simulink model "DigitalControl"  (R2026b)
settings: Solver=VariableStepAuto  MaxStep=0.1  EnableMultiTasking=on
undefined symbols (not defined in the file): deltat, deltat1, DiscIntNeverNeededParam, fden, fnum, Ka, Kf, Ki, Kq, Tal, Ts, W1, W2
libraries: simulink x1
settings Model: DataDictionary=controller.sldd  FPTRunName=Active  ModifiedByFormat=The MathWorks Inc.  Creator=The MathWorks, Inc.  LastModifiedBy=The MathWorks Inc.
settings DataIOCC: LimitDataPoints=on  ReturnWorkspaceOutputs=off  SaveFormat=Array  SaveOutput=off  SaveTime=off  SignalLogging=off  SignalLoggingName=DigitalControl
settings OptimizationCC: LifeSpan=inf  MemsetInitFltsAndDblsToZero=off
settings DebuggingCC: AllowSymbolicDim=off  ArithmeticOperatorsInVariantConditions=warning  FcnCallInpInsideContextMsg=warning  MergeDetectMultiDrivingBlocksExec=none  MultiTaskCondExecSysMsg=none  MultiTaskDSMMsg=warning  SFExecutionAtInitializationDiag=none  SFNoUnconditionalDefaultTransitionDiag=warning  SFUnexpectedBacktrackingDiag=warning  SaveWithParameterizedLinksMsg=none  SignalResolutionControl=TryResolveAllWithWarning  SolverPrmCheckMsg=warning  StateNameClashWarn=warning  UnderspecifiedInitializationDetection=Classic
settings HardwareCC: ProdEndianess=Unspecified  ProdHWDeviceType=32-bit Generic  ProdIntDivRoundTo=Undefined  ProdLargestAtomicFloat=None
settings ModelReferenceCC: ModelReferenceMinAlgLoopOccurrences=on  PropagateSignalLabelsOutOfModel=off
settings SFSimCC: CustomCodeUndefinedFunction=UseInterfaceOnly  SimUseLocalCustomCode=off
settings RTWCC: RTWUseLocalCustomCode=off
settings CodeAppCC: StateflowObjectComments=on
settings GRTTargetCC: CombineOutputUpdateFcns=off  GRTInterface=on  TargetFcnLib=ansi_tfl_tmw.mat  TargetLangStandard=C89/C90 (ANSI)
settings ConfigComp: CovExternalEMLEnable=off  CovSFcnEnable=off  CovSaveCumulativeToWorkspaceVar=on  CovSaveSingleToWorkspaceVar=on

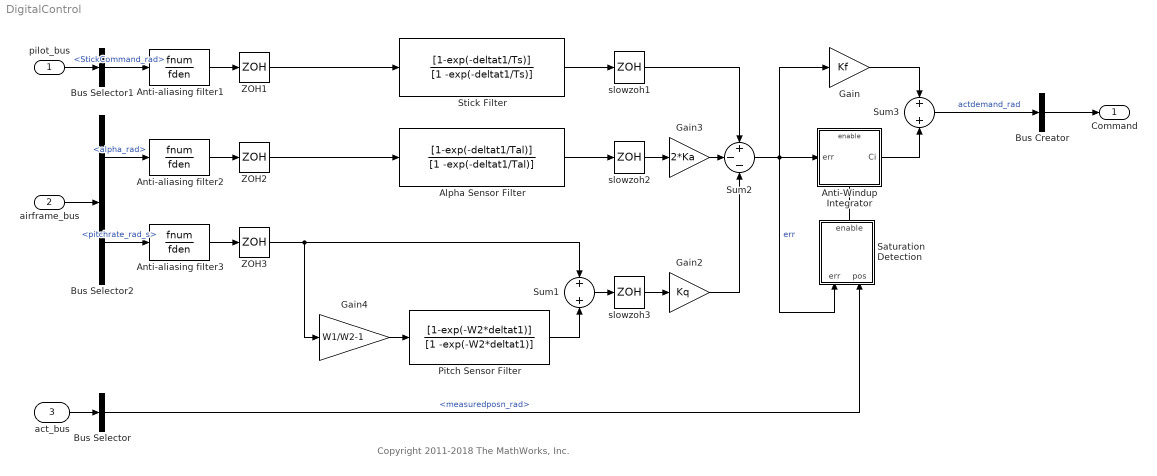
== system DigitalControl ==
  note: Copyright 2011-2018 The MathWorks, Inc.
  pilot_bus : Inport  OutDataTypeStr=Bus: PILOT_BUS
  airframe_bus : Inport  Port=2  OutDataTypeStr=Bus: AIRFRAME_BUS
  act_bus : Inport  Port=3  OutDataTypeStr=Bus: ACT_BUS
  Alpha Sensor Filter : DiscreteTransferFcn  Numerator=[1-exp(-deltat1/Tal)]  Denominator=[1 -exp(-deltat1/Tal)]  SampleTime=deltat1
  Anti-Windup Integrator : Subsystem  TreatAsAtomicUnit=on
      settings: RTWSystemCode=Inline
  Anti-aliasing filter1 : TransferFcn  Numerator=fnum  Denominator=fden
      settings: AttributesFormatString=%<Description>
  Anti-aliasing filter2 : TransferFcn  Numerator=fnum  Denominator=fden
      settings: AttributesFormatString=%<Description>
  Anti-aliasing filter3 : TransferFcn  Numerator=fnum  Denominator=fden
      settings: AttributesFormatString=%<Description>
  Bus Creator : BusCreator  Inputs=1  OutDataTypeStr=Bus: CONTROL_BUS
  Bus Selector : BusSelector  OutputSignals=measuredposn_rad
  Bus Selector1 : BusSelector  OutputSignals=StickCommand_rad
  Bus Selector2 : BusSelector  OutputSignals=alpha_rad,pitchrate_rad_s
  Gain : Gain  Gain=Kf  SaturateOnIntegerOverflow=on  OutDataTypeStr=Inherit: Same as input  ParamDataTypeStr=Inherit: Same as input
  Gain2 : Gain  Gain=Kq  SaturateOnIntegerOverflow=on  OutDataTypeStr=Inherit: Same as input  ParamDataTypeStr=Inherit: Same as input
  Gain3 : Gain  Gain=2*Ka  SaturateOnIntegerOverflow=on  OutDataTypeStr=Inherit: Same as input  ParamDataTypeStr=Inherit: Same as input
  Gain4 : Gain  Gain=W1/W2-1  SaturateOnIntegerOverflow=on  OutDataTypeStr=Inherit: Same as input  ParamDataTypeStr=Inherit: Same as input
  Pitch Sensor Filter : DiscreteTransferFcn  Numerator=[1-exp(-W2*deltat1)]  Denominator=[1 -exp(-W2*deltat1)]  SampleTime=deltat1
  Saturation Detection : Subsystem
  Stick Filter : DiscreteTransferFcn  Numerator=[1-exp(-deltat1/Ts)]  Denominator=[1 -exp(-deltat1/Ts)]  SampleTime=deltat1
  Sum1 : Sum  Inputs=2  InputSameDT=on  SaturateOnIntegerOverflow=on  OutDataTypeStr=Inherit: Same as first input
  Sum2 : Sum  Inputs=+--  InputSameDT=on  SaturateOnIntegerOverflow=on  OutDataTypeStr=Inherit: Same as first input
  Sum3 : Sum  Inputs=2  InputSameDT=on  SaturateOnIntegerOverflow=on  OutDataTypeStr=Inherit: Same as first input
  ZOH1 : ZeroOrderHold  SampleTime=deltat1
  ZOH2 : ZeroOrderHold  SampleTime=deltat1
  ZOH3 : ZeroOrderHold  SampleTime=deltat1
  slowzoh1 : ZeroOrderHold  SampleTime=deltat
  slowzoh2 : ZeroOrderHold  SampleTime=deltat
  slowzoh3 : ZeroOrderHold  SampleTime=deltat
  Command : Outport  OutDataTypeStr=Bus: CONTROL_BUS  VectorParamsAs1DForOutWhenUnconnected=off
  wires:
  pilot_bus/1 -> Bus Selector1/1
  act_bus/1 -> Bus Selector/1
  airframe_bus/1 -> Bus Selector2/1
  Bus Creator/1 -> Command/1
  Bus Selector/1 -> Saturation Detection/2(pos)  "<measuredposn_rad>"
  Saturation Detection/1(enable) -> Anti-Windup Integrator/Enable
  ZOH3/1 -> Sum1/1, Gain4/1
  ZOH2/1 -> Alpha Sensor Filter/1
  Anti-aliasing filter3/1 -> ZOH3/1
  Anti-aliasing filter2/1 -> ZOH2/1
  Anti-aliasing filter1/1 -> ZOH1/1
  ZOH1/1 -> Stick Filter/1
  Bus Selector1/1 -> Anti-aliasing filter1/1  "<StickCommand_rad>"
  slowzoh3/1 -> Gain2/1
  Gain4/1 -> Pitch Sensor Filter/1
  Pitch Sensor Filter/1 -> Sum1/2
  Sum1/1 -> slowzoh3/1
  Bus Selector2/2 -> Anti-aliasing filter3/1  "<pitchrate_rad_s>"
  Gain2/1 -> Sum2/3
  Anti-Windup Integrator/1(Ci) -> Sum3/2
  Gain/1 -> Sum3/1
  Gain3/1 -> Sum2/2
  slowzoh2/1 -> Gain3/1
  Alpha Sensor Filter/1 -> slowzoh2/1
  slowzoh1/1 -> Sum2/1
  Stick Filter/1 -> slowzoh1/1
  Bus Selector2/1 -> Anti-aliasing filter2/1  "<alpha_rad>"
  Sum2/1 -> Gain/1, Anti-Windup Integrator/1(err), Saturation Detection/1(err)  "err"
  Sum3/1 -> Bus Creator/1  "actdemand_rad"

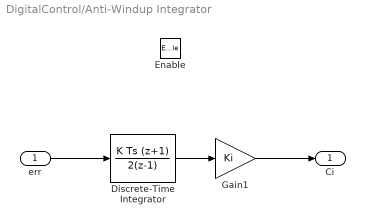
== system DigitalControl/Anti-Windup Integrator ==
  err : Inport
  Enable : EnablePort
  Discrete-Time Integrator : DiscreteIntegrator  IntegratorMethod=Integration: Trapezoidal  SampleTime=deltat  ICPrevOutput=DiscIntNeverNeededParam  ICPrevScaledInput=DiscIntNeverNeededParam
  Gain1 : Gain  Gain=Ki  SaturateOnIntegerOverflow=on  OutDataTypeStr=Inherit: Same as input  ParamDataTypeStr=Inherit: Same as input
  Ci : Outport  InitialOutput=0  VectorParamsAs1DForOutWhenUnconnected=off
  wires:
  err/1 -> Discrete-Time Integrator/1
  Discrete-Time Integrator/1 -> Gain1/1
  Gain1/1 -> Ci/1

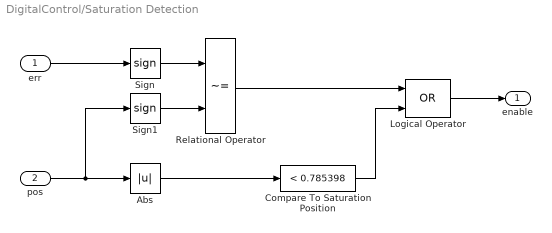
== system DigitalControl/Saturation Detection ==
  err : Inport
  pos : Inport  Port=2
  Abs : Abs  ZeroCross=off  SaturateOnIntegerOverflow=off
  Compare To Saturation Position : simulink/Logic and Bit Operations/Compare To Constant  relop=<  const=0.785398  OutDataTypeStr=boolean  ZeroCross=off
  Logical Operator : Logic  Operator=OR  AllPortsSameDT=off  OutDataTypeStr=boolean
  Relational Operator : RelationalOperator  Operator=~=  OutDataTypeStr=boolean  ZeroCross=off  InputSameDT=off
  Sign : Signum  ZeroCross=off
  Sign1 : Signum  ZeroCross=off
  enable : Outport  VectorParamsAs1DForOutWhenUnconnected=off
  wires:
  pos/1 -> Sign1/1, Abs/1
  Sign/1 -> Relational Operator/1
  Relational Operator/1 -> Logical Operator/1
  Compare To Saturation Position/1 -> Logical Operator/2
  Sign1/1 -> Relational Operator/2
  Abs/1 -> Compare To Saturation Position/1
  err/1 -> Sign/1
  Logical Operator/1 -> enable/1
